simulink model "Drone_Sim_clean"  (R2018b)
settings: Solver=ode15s  StartTime=0.0  StopTime=50  FixedStep=0.1
model workspace (MAT data in the model file):
  A_matrix = [0  0  0  0  0  0  1  0  0  0  0  0; 0  0  0  0  0  0  0  1  0  0  0  0; 0  0  0  0  0  0  0  0  1  0  0  0; 0  0  0  0  0  0  0  0  0  1  0  0; 0  0  0  0  0  0  0  0  0  0  1  0; 0  0  0  0  0  0  0  0  0  0  0  1; 0  0  0  0  9.81  0  0  0  0  0  0  0; 0  0  0  0  0  -9.81  0  0  0  0  0  0; 0  0  0  0  0  0  0  0  0  0  0  0; 0  0  0  0  0  0  0  0  0  0  0  0; 0  0  0  0  0  0  0  0  0  0  0  0; 0  0  0  0  0  0  0  0  0  0  0  0]
values from neighbouring files (symbols this model uses):
  A = [ 0 0 0 0 0 0 1 0 0 0 0 0 ... (first row only)    [A_and_B_for_drone_system_dynamics_simulink.m]
  B = we .* [ 0 0 0 0 ... (first row only)    [A_and_B_for_drone_system_dynamics_simulink.m]
  C = eye(12)    [A_and_B_for_drone_system_dynamics_simulink.m]
  D = zeros(12,4)    [A_and_B_for_drone_system_dynamics_simulink.m]
libraries: simulink x7
settings Model: EnablePacing=on  Creator=harry  LastModifiedBy=Chris

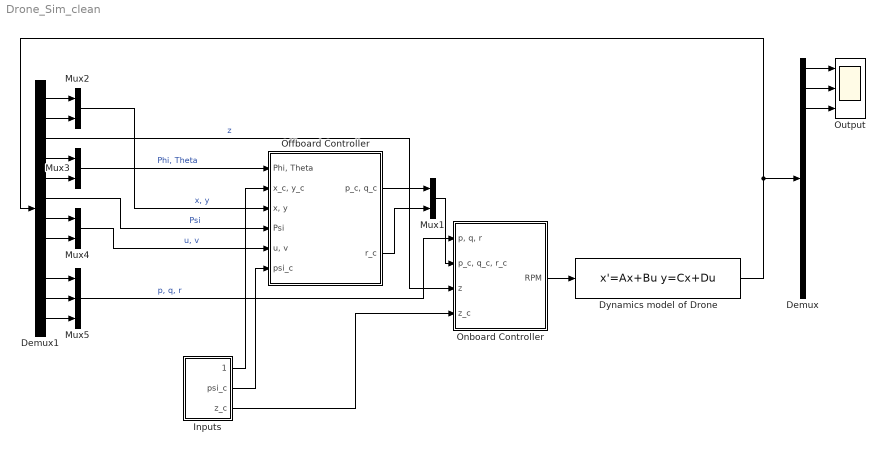
== system Drone_Sim_clean ==
  Demux : Demux  Outputs=12
  Demux1 : Demux  Outputs=12
  Dynamics model of Drone : StateSpace  A=A  B=B  C=C  D=D  InitialCondition=[0,0,0,0,0,0,0,0,0,0,0,0]  ContinuousStateAttributes='X.Y.Z.Roll.PItch.Yaw.U.V.W.Roll_Rate.Pitch_Rate.Yaw_Rate'
  Inputs : Subsystem
  Mux{1..4} (4 alike) : Mux  Inputs=2
  Mux5 : Mux  Inputs=3
  Offboard Controller : Subsystem
  Onboard Controller : Subsystem
  Output : Scope  NumInputPorts=3
  wires:
  Demux1/1 -> Mux2/1
  Demux1/2 -> Mux2/2
  Demux1/5 -> Mux3/2
  Demux1/6 -> Offboard Controller/4(Psi)  "Psi"
  Demux1/7 -> Mux4/1
  Demux1/8 -> Mux4/2
  Demux1/12 -> Mux5/3
  Demux1/11 -> Mux5/2
  Demux1/10 -> Mux5/1
  Demux/2 -> Output/2
  Mux2/1 -> Offboard Controller/3("x, y ")  "x, y"
  Mux3/1 -> Offboard Controller/1("Phi, Theta")  "Phi, Theta"
  Demux1/4 -> Mux3/1
  Mux4/1 -> Offboard Controller/5("u, v ")  "u, v"
  Inputs/1("x_c, y_c") -> Offboard Controller/2("x_c, y_c")
  Inputs/2(psi_c) -> Offboard Controller/6(psi_c)
  Offboard Controller/1("p_c, q_c") -> Mux1/1
  Offboard Controller/2(r_c) -> Mux1/2
  Mux5/1 -> Onboard Controller/1("p, q, r")  "p, q, r"
  Demux1/3 -> Onboard Controller/3(z)  "z"
  Mux1/1 -> Onboard Controller/2("p_c, q_c, r_c")
  Inputs/3(z_c) -> Onboard Controller/4(z_c)
  Onboard Controller/1(RPM) -> Dynamics model of Drone/1
  Dynamics model of Drone/1 -> Demux/1, Demux1/1
  Demux/1 -> Output/1
  Demux/3 -> Output/3

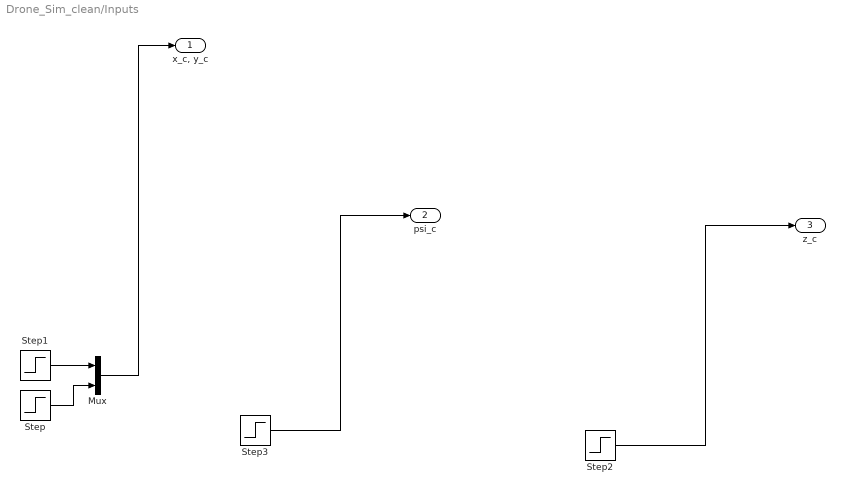
== system Drone_Sim_clean/Inputs ==
  Mux : Mux  Inputs=2
  Step : Step  After=0.3  SampleTime=0
  Step1 : Step  After=0.3  SampleTime=0
  Step2 : Step  After=0.3  SampleTime=0
  Step3 : Step  After=0  SampleTime=0
  "x_c, y_c" : Outport
  psi_c : Outport  Port=2
  z_c : Outport  Port=3
  wires:
  Step1/1 -> Mux/1
  Step2/1 -> z_c/1
  Step3/1 -> psi_c/1
  Mux/1 -> "x_c, y_c"/1
  Step/1 -> Mux/2

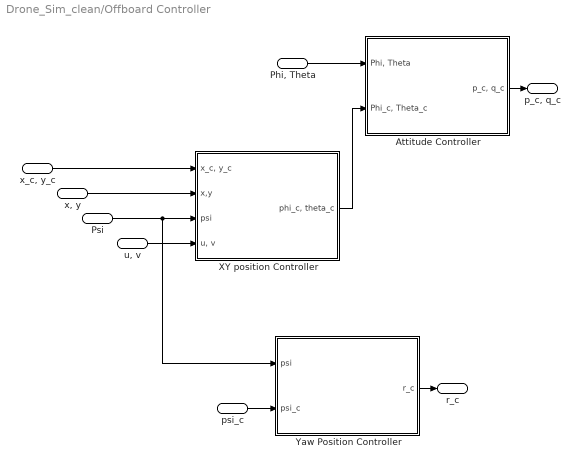
== system Drone_Sim_clean/Offboard Controller ==
  "Phi, Theta" : Inport
  "x_c, y_c" : Inport  Port=2
  "x, y " : Inport  Port=3
  Psi : Inport  Port=4
  "u, v " : Inport  Port=5
  psi_c : Inport  Port=6
  Attitude Controller : Subsystem
  XY position Controller : Subsystem
  "Yaw Position Controller " : Subsystem
  "p_c, q_c" : Outport
  r_c : Outport  Port=2
  wires:
  "u, v "/1 -> XY position Controller/4("u, v")
  "Yaw Position Controller "/1(r_c) -> r_c/1
  XY position Controller/1("phi_c, theta_c") -> Attitude Controller/2("Phi_c, Theta_c")
  Attitude Controller/1("p_c, q_c") -> "p_c, q_c"/1
  "x, y "/1 -> XY position Controller/2(x,y)
  "Phi, Theta"/1 -> Attitude Controller/1("Phi, Theta")
  "x_c, y_c"/1 -> XY position Controller/1("x_c, y_c")
  psi_c/1 -> "Yaw Position Controller "/2(psi_c)
  Psi/1 -> "Yaw Position Controller "/1(psi), XY position Controller/3(psi)

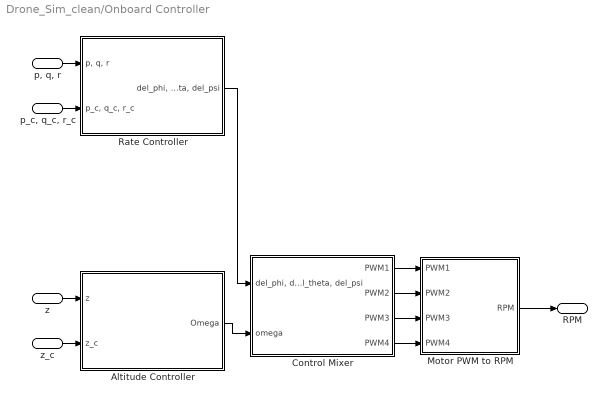
== system Drone_Sim_clean/Onboard Controller ==
  "p, q, r" : Inport
  "p_c, q_c, r_c" : Inport  Port=2
  z : Inport  Port=3
  z_c : Inport  Port=4
  Altitude Controller : Subsystem
  Control Mixer : Subsystem
  Motor PWM to RPM : Subsystem
  Rate Controller : Subsystem
  RPM : Outport
  wires:
  z_c/1 -> Altitude Controller/2(z_c)
  "p_c, q_c, r_c"/1 -> Rate Controller/2("p_c, q_c, r_c")
  Control Mixer/1("PWM1 ") -> Motor PWM to RPM/1(PWM1)
  "p, q, r"/1 -> Rate Controller/1("p, q, r")
  z/1 -> Altitude Controller/1(z)
  Motor PWM to RPM/1("RPM ") -> RPM/1
  Rate Controller/1("del_phi, del_theta, del_psi") -> Control Mixer/1("del_phi, del_theta, del_psi")
  Control Mixer/2("PWM2 ") -> Motor PWM to RPM/2(PWM2)
  Control Mixer/3(PWM3) -> Motor PWM to RPM/3(PWM3)
  Control Mixer/4("PWM4 ") -> Motor PWM to RPM/4("PWM4 ")
  Altitude Controller/1(Omega) -> Control Mixer/2("omega ")

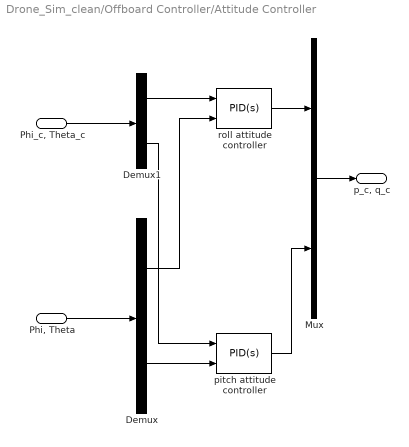
== system Drone_Sim_clean/Offboard Controller/Attitude Controller ==
  "Phi, Theta" : Inport
  "Phi_c, Theta_c" : Inport  Port=2
  Demux : Demux  Outputs=2
  Demux1 : Demux  Outputs=2
  Mux : Mux  Inputs=2
  pitch attitude controller : simulink/Continuous/PID Controller (2DOF)  Controller=PID  Form=Parallel  TimeDomain=Continuous-time  SampleTime=-1  IntegratorMethod=Forward Euler  FilterMethod=Forward Euler  ControllerParametersSource=internal  P=3.5  I=2  D=0  UseFilter=on  N=100  b=1  c=1  TunerSelectOption=Transfer Function Based (PID Tuner App)  InitialConditionSource=internal  InitialConditionForIntegrator=0  InitialConditionForFilter=0  DifferentiatorICPrevScaledInput=0  ExternalReset=none  TrackingMode=off  Kt=1  LimitOutput=on  UpperSaturationLimit=0.5  LowerSaturationLimit=-0.5  LinearizeAsGain=off  AntiWindupMode=clamping  Kb=1  POutMin=[]  POutMax=[]  IOutMin=[]  IOutMax=[]  DOutMin=[]  DOutMax=[]  NOutMin=[]  NOutMax=[]  bOutMin=[]  bOutMax=[]  cOutMin=[]  cOutMax=[]  SumOutMin=[]  SumOutMax=[]  SaturationOutMin=[]  SaturationOutMax=[]  PParamMin=[]  PParamMax=[]  IParamMin=[]  IParamMax=[]  DParamMin=[]  DParamMax=[]  NParamMin=[]  NParamMax=[]  bParamMin=[]  bParamMax=[]  cParamMin=[]  cParamMax=[]  KbParamMin=[]  KbParamMax=[]  KtParamMin=[]  KtParamMax=[]  KbOutMin=[]  KbOutMax=[]  KtOutMin=[]  KtOutMax=[]  IntegratorOutMin=[]  IntegratorOutMax=[]  FilterOutMin=[]  FilterOutMax=[]  SumI1OutMin=[]  SumI1OutMax=[]  SumI2OutMin=[]  SumI2OutMax=[]  SumI3OutMin=[]  SumI3OutMax=[]  SumI4OutMin=[]  SumI4OutMax=[]  SumDOutMin=[]  SumDOutMax=[]  Sum1OutMin=[]  Sum1OutMax=[]  Sum2OutMin=[]  Sum2OutMax=[]  Sum3OutMin=[]  Sum3OutMax=[]  DifferentiatorOutMin=[]  DifferentiatorOutMax=[]  FilterDiffOutCoefMin=[]  FilterDiffOutCoefMax=[]  ReciprocalOutMin=[]  ReciprocalOutMax=[]  SumDenOutMin=[]  SumDenOutMax=[]  SumNumOutMin=[]  SumNumOutMax=[]  DivideOutMin=[]  DivideOutMax=[]  IntegratorContinuousStateAttributes=''  IntegratorStateMustResolveToSignalObject=off  IntegratorRTWStateStorageClass=Auto  FilterContinuousStateAttributes=''  FilterStateMustResolveToSignalObject=off  FilterRTWStateStorageClass=Auto  ParallelPVariant=InternalParameters  IdealPVariant=Disabled  IVariant=InternalParameters  DVariant=InternalParameters  bVariant=InternalParameters  cVariant=InternalParameters  IntegratorVariant=Continuous  SatVariant=Enabled  AWVariant=ContClampingParallel  PCopyVariant=Disabled  TRVariant=Disabled  FdbkBlocksVariant=Forward  IdealPFdbkVariant=Disabled  SatFdbkVariant=Disabled  DerivativeFilterVariant=ContFilter  NVariant=InternalParameters  NCopyVariant=Disabled  FilterICVariant=InternalICsFilter  IntegratorICVariant=InternalICs  ExternalResetVariant=Disabled  TRSumVariant=Passthrough  SumFdbkVariant=Disabled  SumVariant=Sum_PID
  roll attitude controller : simulink/Continuous/PID Controller (2DOF)  Controller=PID  Form=Parallel  TimeDomain=Continuous-time  SampleTime=-1  IntegratorMethod=Forward Euler  FilterMethod=Forward Euler  ControllerParametersSource=internal  P=3.5  I=2  D=0  UseFilter=on  N=100  b=1  c=1  TunerSelectOption=Transfer Function Based (PID Tuner App)  InitialConditionSource=internal  InitialConditionForIntegrator=0  InitialConditionForFilter=0  DifferentiatorICPrevScaledInput=0  ExternalReset=none  TrackingMode=off  Kt=1  LimitOutput=on  UpperSaturationLimit=0.5  LowerSaturationLimit=-0.5  LinearizeAsGain=off  AntiWindupMode=clamping  Kb=1  POutMin=[]  POutMax=[]  IOutMin=[]  IOutMax=[]  DOutMin=[]  DOutMax=[]  NOutMin=[]  NOutMax=[]  bOutMin=[]  bOutMax=[]  cOutMin=[]  cOutMax=[]  SumOutMin=[]  SumOutMax=[]  SaturationOutMin=[]  SaturationOutMax=[]  PParamMin=[]  PParamMax=[]  IParamMin=[]  IParamMax=[]  DParamMin=[]  DParamMax=[]  NParamMin=[]  NParamMax=[]  bParamMin=[]  bParamMax=[]  cParamMin=[]  cParamMax=[]  KbParamMin=[]  KbParamMax=[]  KtParamMin=[]  KtParamMax=[]  KbOutMin=[]  KbOutMax=[]  KtOutMin=[]  KtOutMax=[]  IntegratorOutMin=[]  IntegratorOutMax=[]  FilterOutMin=[]  FilterOutMax=[]  SumI1OutMin=[]  SumI1OutMax=[]  SumI2OutMin=[]  SumI2OutMax=[]  SumI3OutMin=[]  SumI3OutMax=[]  SumI4OutMin=[]  SumI4OutMax=[]  SumDOutMin=[]  SumDOutMax=[]  Sum1OutMin=[]  Sum1OutMax=[]  Sum2OutMin=[]  Sum2OutMax=[]  Sum3OutMin=[]  Sum3OutMax=[]  DifferentiatorOutMin=[]  DifferentiatorOutMax=[]  FilterDiffOutCoefMin=[]  FilterDiffOutCoefMax=[]  ReciprocalOutMin=[]  ReciprocalOutMax=[]  SumDenOutMin=[]  SumDenOutMax=[]  SumNumOutMin=[]  SumNumOutMax=[]  DivideOutMin=[]  DivideOutMax=[]  IntegratorContinuousStateAttributes=''  IntegratorStateMustResolveToSignalObject=off  IntegratorRTWStateStorageClass=Auto  FilterContinuousStateAttributes=''  FilterStateMustResolveToSignalObject=off  FilterRTWStateStorageClass=Auto  ParallelPVariant=InternalParameters  IdealPVariant=Disabled  IVariant=InternalParameters  DVariant=InternalParameters  bVariant=InternalParameters  cVariant=InternalParameters  IntegratorVariant=Continuous  SatVariant=Enabled  AWVariant=ContClampingParallel  PCopyVariant=Disabled  TRVariant=Disabled  FdbkBlocksVariant=Forward  IdealPFdbkVariant=Disabled  SatFdbkVariant=Disabled  DerivativeFilterVariant=ContFilter  NVariant=InternalParameters  NCopyVariant=Disabled  FilterICVariant=InternalICsFilter  IntegratorICVariant=InternalICs  ExternalResetVariant=Disabled  TRSumVariant=Passthrough  SumFdbkVariant=Disabled  SumVariant=Sum_PID
  "p_c, q_c" : Outport  VectorParamsAs1DForOutWhenUnconnected=off
  wires:
  "Phi, Theta"/1 -> Demux/1
  "Phi_c, Theta_c"/1 -> Demux1/1
  Mux/1 -> "p_c, q_c"/1
  Demux1/1 -> roll attitude controller/1
  Demux/1 -> roll attitude controller/2
  roll attitude controller/1 -> Mux/1
  Demux/2 -> pitch attitude controller/2
  Demux1/2 -> pitch attitude controller/1
  pitch attitude controller/1 -> Mux/2

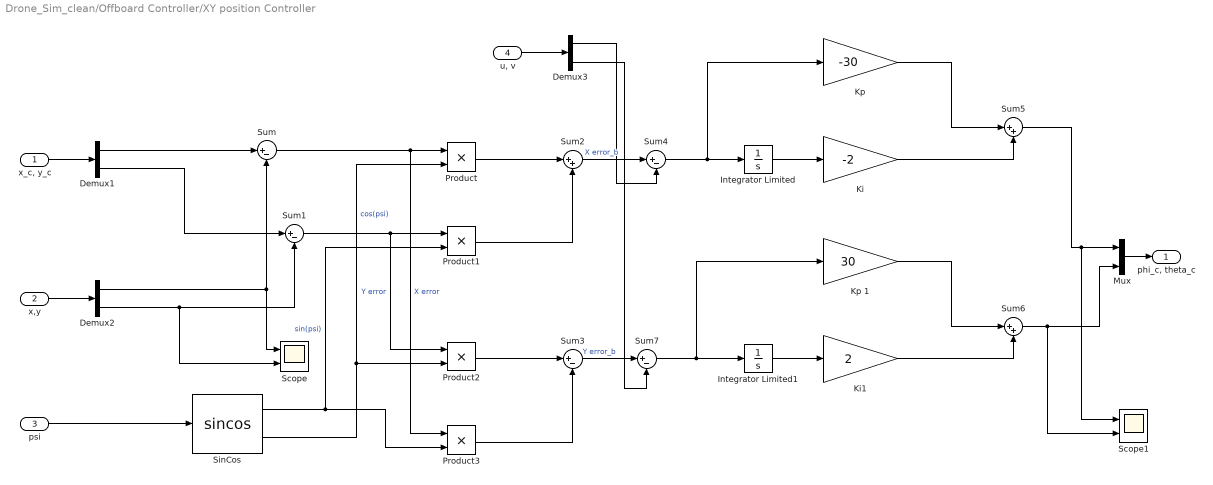
== system Drone_Sim_clean/Offboard Controller/XY position Controller ==
  "x_c, y_c" : Inport
  x,y : Inport  Port=2
  psi : Inport  Port=3
  "u, v" : Inport  Port=4
  Demux1 : Demux  Outputs=2
  Demux2 : Demux  Outputs=2
  Demux3 : Demux  Outputs=2
  Integrator Limited : Integrator  LimitOutput=on  UpperSaturationLimit=pi/6  LowerSaturationLimit=-pi/6
  Integrator Limited1 : Integrator  LimitOutput=on  UpperSaturationLimit=pi/6  LowerSaturationLimit=-pi/6
  Ki : Gain  Gain=-2
  Ki1 : Gain  Gain=2
  "Kp " : Gain  Gain=-30
  Kp 1 : Gain  Gain=30
  Mux : Mux  Inputs=2
  Product{,1..3} (4 alike) : Product
  Scope : Scope  NumInputPorts=2
  Scope1 : Scope  NumInputPorts=2
  SinCos : Trigonometry  Operator=sincos
  Sum{,1,3..4,7} (5 alike) : Sum  Inputs=|+-
  Sum2 : Sum  Inputs=|++
  Sum5 : Sum  Inputs=|++
  Sum6 : Sum  Inputs=|++
  "phi_c, theta_c" : Outport  VectorParamsAs1DForOutWhenUnconnected=off
  wires:
  "x_c, y_c"/1 -> Demux1/1
  x,y/1 -> Demux2/1
  "u, v"/1 -> Demux3/1
  Demux1/1 -> Sum/1
  Demux2/1 -> Scope/1, Sum/2
  Sum/1 -> Product3/1, Product/1  "X error"
  psi/1 -> SinCos/1
  SinCos/2 -> Product2/2, Product/2  "cos(psi)"
  Demux1/2 -> Sum1/1
  Demux2/2 -> Scope/2, Sum1/2
  Sum1/1 -> Product2/1, Product1/1  "Y error"
  SinCos/1 -> Product1/2, Product3/2  "sin(psi)"
  Product/1 -> Sum2/1
  Product1/1 -> Sum2/2
  Product2/1 -> Sum3/1
  Product3/1 -> Sum3/2
  Sum2/1 -> Sum4/1  "X error_b"
  Demux3/1 -> Sum4/2
  Sum4/1 -> "Kp "/1, Integrator Limited/1
  Integrator Limited/1 -> Ki/1
  Integrator Limited1/1 -> Ki1/1
  "Kp "/1 -> Sum5/1
  Ki/1 -> Sum5/2
  Ki1/1 -> Sum6/2
  Kp 1/1 -> Sum6/1
  Mux/1 -> "phi_c, theta_c"/1
  Sum3/1 -> Sum7/1  "Y error_b"
  Demux3/2 -> Sum7/2
  Sum7/1 -> Kp 1/1, Integrator Limited1/1
  Sum5/1 -> Scope1/1, Mux/1
  Sum6/1 -> Scope1/2, Mux/2

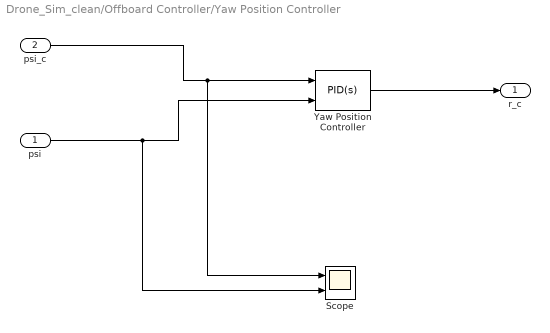
== system Drone_Sim_clean/Offboard Controller/Yaw Position Controller  ==
  psi : Inport
  psi_c : Inport  Port=2
  Scope : Scope  NumInputPorts=2
  Yaw Position Controller : simulink/Continuous/PID Controller (2DOF)  Controller=PID  Form=Parallel  TimeDomain=Continuous-time  SampleTime=-1  IntegratorMethod=Forward Euler  FilterMethod=Forward Euler  ControllerParametersSource=internal  P=3  I=0  D=0  UseFilter=on  N=100  b=1  c=1  TunerSelectOption=Transfer Function Based (PID Tuner App)  InitialConditionSource=internal  InitialConditionForIntegrator=0  InitialConditionForFilter=0  DifferentiatorICPrevScaledInput=0  ExternalReset=none  TrackingMode=off  Kt=1  LimitOutput=on  UpperSaturationLimit=1  LowerSaturationLimit=-1  LinearizeAsGain=on  AntiWindupMode=none  Kb=1  POutMin=[]  POutMax=[]  IOutMin=[]  IOutMax=[]  DOutMin=[]  DOutMax=[]  NOutMin=[]  NOutMax=[]  bOutMin=[]  bOutMax=[]  cOutMin=[]  cOutMax=[]  SumOutMin=[]  SumOutMax=[]  SaturationOutMin=[]  SaturationOutMax=[]  PParamMin=[]  PParamMax=[]  IParamMin=[]  IParamMax=[]  DParamMin=[]  DParamMax=[]  NParamMin=[]  NParamMax=[]  bParamMin=[]  bParamMax=[]  cParamMin=[]  cParamMax=[]  KbParamMin=[]  KbParamMax=[]  KtParamMin=[]  KtParamMax=[]  KbOutMin=[]  KbOutMax=[]  KtOutMin=[]  KtOutMax=[]  IntegratorOutMin=[]  IntegratorOutMax=[]  FilterOutMin=[]  FilterOutMax=[]  SumI1OutMin=[]  SumI1OutMax=[]  SumI2OutMin=[]  SumI2OutMax=[]  SumI3OutMin=[]  SumI3OutMax=[]  SumI4OutMin=[]  SumI4OutMax=[]  SumDOutMin=[]  SumDOutMax=[]  Sum1OutMin=[]  Sum1OutMax=[]  Sum2OutMin=[]  Sum2OutMax=[]  Sum3OutMin=[]  Sum3OutMax=[]  DifferentiatorOutMin=[]  DifferentiatorOutMax=[]  FilterDiffOutCoefMin=[]  FilterDiffOutCoefMax=[]  ReciprocalOutMin=[]  ReciprocalOutMax=[]  SumDenOutMin=[]  SumDenOutMax=[]  SumNumOutMin=[]  SumNumOutMax=[]  DivideOutMin=[]  DivideOutMax=[]  IntegratorContinuousStateAttributes=''  IntegratorStateMustResolveToSignalObject=off  IntegratorRTWStateStorageClass=Auto  FilterContinuousStateAttributes=''  FilterStateMustResolveToSignalObject=off  FilterRTWStateStorageClass=Auto  ParallelPVariant=InternalParameters  IdealPVariant=Disabled  IVariant=InternalParameters  DVariant=InternalParameters  bVariant=InternalParameters  cVariant=InternalParameters  IntegratorVariant=Continuous  SatVariant=Enabled  AWVariant=Passthrough  PCopyVariant=Disabled  TRVariant=Disabled  FdbkBlocksVariant=Forward  IdealPFdbkVariant=Disabled  SatFdbkVariant=Disabled  DerivativeFilterVariant=ContFilter  NVariant=InternalParameters  NCopyVariant=Disabled  FilterICVariant=InternalICsFilter  IntegratorICVariant=InternalICs  ExternalResetVariant=Disabled  TRSumVariant=Passthrough  SumFdbkVariant=Disabled  SumVariant=Sum_PID
  r_c : Outport  VectorParamsAs1DForOutWhenUnconnected=off
  wires:
  psi/1 -> Scope/2, Yaw Position Controller/2
  psi_c/1 -> Scope/1, Yaw Position Controller/1
  Yaw Position Controller/1 -> r_c/1

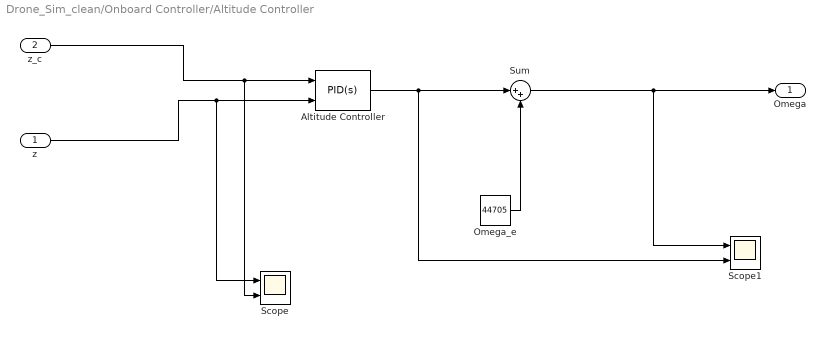
== system Drone_Sim_clean/Onboard Controller/Altitude Controller ==
  z : Inport
  z_c : Inport  Port=2
  Altitude Controller : simulink/Continuous/PID Controller (2DOF)  Controller=PID  Form=Parallel  TimeDomain=Continuous-time  SampleTime=-1  IntegratorMethod=Forward Euler  FilterMethod=Forward Euler  ControllerParametersSource=internal  P=11000  I=3500  D=9000  UseFilter=on  N=100  b=1  c=1  TunerSelectOption=Transfer Function Based (PID Tuner App)  InitialConditionSource=internal  InitialConditionForIntegrator=0  InitialConditionForFilter=0  DifferentiatorICPrevScaledInput=0  ExternalReset=none  TrackingMode=off  Kt=1  LimitOutput=on  UpperSaturationLimit=15000  LowerSaturationLimit=-20000  LinearizeAsGain=on  AntiWindupMode=clamping  Kb=1  POutMin=[]  POutMax=[]  IOutMin=[]  IOutMax=[]  DOutMin=[]  DOutMax=[]  NOutMin=[]  NOutMax=[]  bOutMin=[]  bOutMax=[]  cOutMin=[]  cOutMax=[]  SumOutMin=[]  SumOutMax=[]  SaturationOutMin=[]  SaturationOutMax=[]  PParamMin=[]  PParamMax=[]  IParamMin=[]  IParamMax=[]  DParamMin=[]  DParamMax=[]  NParamMin=[]  NParamMax=[]  bParamMin=[]  bParamMax=[]  cParamMin=[]  cParamMax=[]  KbParamMin=[]  KbParamMax=[]  KtParamMin=[]  KtParamMax=[]  KbOutMin=[]  KbOutMax=[]  KtOutMin=[]  KtOutMax=[]  IntegratorOutMin=[]  IntegratorOutMax=[]  FilterOutMin=[]  FilterOutMax=[]  SumI1OutMin=[]  SumI1OutMax=[]  SumI2OutMin=[]  SumI2OutMax=[]  SumI3OutMin=[]  SumI3OutMax=[]  SumI4OutMin=[]  SumI4OutMax=[]  SumDOutMin=[]  SumDOutMax=[]  Sum1OutMin=[]  Sum1OutMax=[]  Sum2OutMin=[]  Sum2OutMax=[]  Sum3OutMin=[]  Sum3OutMax=[]  DifferentiatorOutMin=[]  DifferentiatorOutMax=[]  FilterDiffOutCoefMin=[]  FilterDiffOutCoefMax=[]  ReciprocalOutMin=[]  ReciprocalOutMax=[]  SumDenOutMin=[]  SumDenOutMax=[]  SumNumOutMin=[]  SumNumOutMax=[]  DivideOutMin=[]  DivideOutMax=[]  IntegratorContinuousStateAttributes=''  IntegratorStateMustResolveToSignalObject=off  IntegratorRTWStateStorageClass=Auto  FilterContinuousStateAttributes=''  FilterStateMustResolveToSignalObject=off  FilterRTWStateStorageClass=Auto  ParallelPVariant=InternalParameters  IdealPVariant=Disabled  IVariant=InternalParameters  DVariant=InternalParameters  bVariant=InternalParameters  cVariant=InternalParameters  IntegratorVariant=Continuous  SatVariant=Enabled  AWVariant=ContClampingParallel  PCopyVariant=Disabled  TRVariant=Disabled  FdbkBlocksVariant=Forward  IdealPFdbkVariant=Disabled  SatFdbkVariant=Disabled  DerivativeFilterVariant=ContFilter  NVariant=InternalParameters  NCopyVariant=Disabled  FilterICVariant=InternalICsFilter  IntegratorICVariant=InternalICs  ExternalResetVariant=Disabled  TRSumVariant=Passthrough  SumFdbkVariant=Disabled  SumVariant=Sum_PID
  Omega_e : Constant  Value=44705
  Scope : Scope  NumInputPorts=2
  Scope1 : Scope  NumInputPorts=2
  Sum : Sum  Inputs=|++
  Omega : Outport  VectorParamsAs1DForOutWhenUnconnected=off
  wires:
  z_c/1 -> Scope/2, Altitude Controller/1
  Sum/1 -> Scope1/1, Omega/1
  Altitude Controller/1 -> Scope1/2, Sum/1
  Omega_e/1 -> Sum/2
  z/1 -> Scope/1, Altitude Controller/2

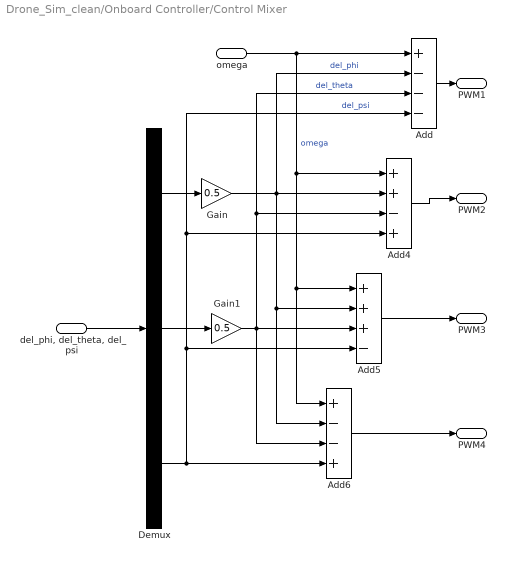
== system Drone_Sim_clean/Onboard Controller/Control Mixer ==
  "del_phi, del_theta, del_psi" : Inport
  "omega " : Inport  Port=2
  Add : Sum  Inputs=+---
  Add4 : Sum  Inputs=++-+
  Add5 : Sum  Inputs=+++-
  Add6 : Sum  Inputs=+--+
  Demux : Demux  Outputs=3
  Gain : Gain  Gain=0.5
  Gain1 : Gain  Gain=0.5
  "PWM1 " : Outport  VectorParamsAs1DForOutWhenUnconnected=off
  "PWM2 " : Outport  Port=2  VectorParamsAs1DForOutWhenUnconnected=off
  PWM3 : Outport  Port=3  VectorParamsAs1DForOutWhenUnconnected=off
  "PWM4 " : Outport  Port=4  VectorParamsAs1DForOutWhenUnconnected=off
  wires:
  "del_phi, del_theta, del_psi"/1 -> Demux/1
  Demux/1 -> Gain/1
  Demux/2 -> Gain1/1
  Add/1 -> "PWM1 "/1
  Add4/1 -> "PWM2 "/1
  Add5/1 -> PWM3/1
  Add6/1 -> "PWM4 "/1
  Demux/3 -> Add/4, Add4/4, Add5/4, Add6/4  "del_psi"
  Gain1/1 -> Add6/3, Add5/3, Add/3, Add4/3  "del_theta"
  Gain/1 -> Add/2, Add4/2, Add6/2, Add5/2  "del_phi"
  "omega "/1 -> Add/1, Add6/1, Add5/1, Add4/1  "omega"

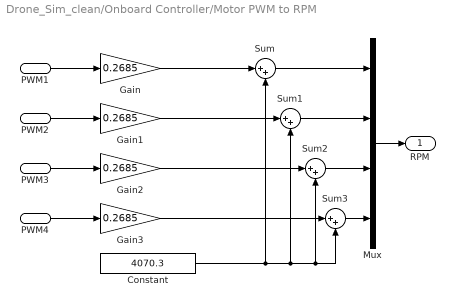
== system Drone_Sim_clean/Onboard Controller/Motor PWM to RPM ==
  PWM1 : Inport
  PWM2 : Inport  Port=2
  PWM3 : Inport  Port=3
  "PWM4 " : Inport  Port=4
  Constant : Constant  Value=4070.3
  Gain{,1..3} (4 alike) : Gain  Gain=0.2685
  Mux : Mux
  Sum{,1..3} (4 alike) : Sum  Inputs=|++
  "RPM " : Outport
  wires:
  Gain/1 -> Sum/1
  PWM1/1 -> Gain/1
  Gain1/1 -> Sum1/1
  Gain2/1 -> Sum2/1
  Gain3/1 -> Sum3/1
  PWM2/1 -> Gain1/1
  PWM3/1 -> Gain2/1
  "PWM4 "/1 -> Gain3/1
  Sum/1 -> Mux/1
  Sum1/1 -> Mux/2
  Sum2/1 -> Mux/3
  Sum3/1 -> Mux/4
  Constant/1 -> Sum/2, Sum3/2, Sum2/2, Sum1/2
  Mux/1 -> "RPM "/1

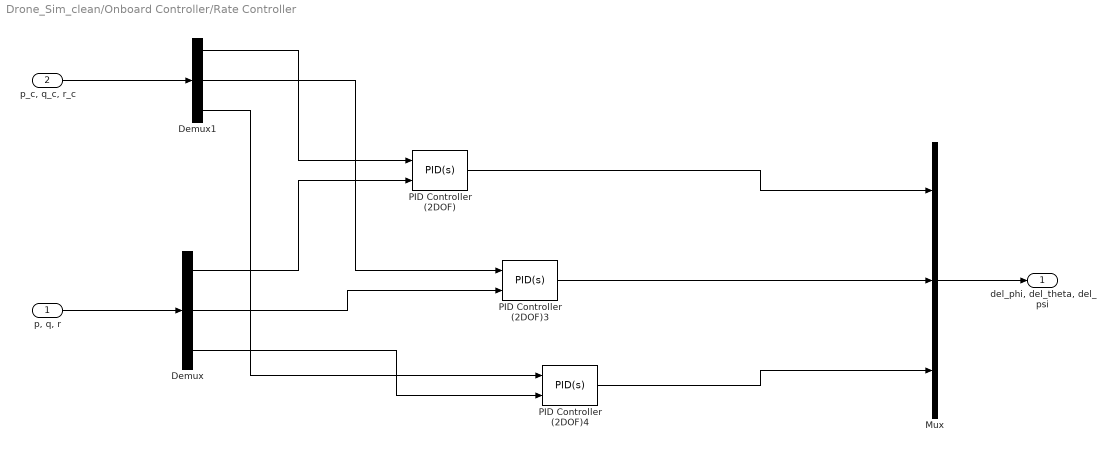
== system Drone_Sim_clean/Onboard Controller/Rate Controller ==
  "p, q, r" : Inport
  "p_c, q_c, r_c" : Inport  Port=2
  Demux : Demux  Outputs=3
  Demux1 : Demux  Outputs=3
  Mux : Mux  Inputs=3
  PID Controller (2DOF) : simulink/Continuous/PID Controller (2DOF)  Controller=PID  Form=Parallel  TimeDomain=Continuous-time  SampleTime=-1  IntegratorMethod=Forward Euler  FilterMethod=Forward Euler  ControllerParametersSource=internal  P=70  I=0  D=0  UseFilter=on  N=100  b=1  c=1  TunerSelectOption=Transfer Function Based (PID Tuner App)  InitialConditionSource=internal  InitialConditionForIntegrator=0  InitialConditionForFilter=0  DifferentiatorICPrevScaledInput=0  ExternalReset=none  TrackingMode=off  Kt=1  LimitOutput=on  UpperSaturationLimit=0.1  LowerSaturationLimit=-0.1  LinearizeAsGain=off  AntiWindupMode=clamping  Kb=1  POutMin=[]  POutMax=[]  IOutMin=[]  IOutMax=[]  DOutMin=[]  DOutMax=[]  NOutMin=[]  NOutMax=[]  bOutMin=[]  bOutMax=[]  cOutMin=[]  cOutMax=[]  SumOutMin=[]  SumOutMax=[]  SaturationOutMin=[]  SaturationOutMax=[]  PParamMin=[]  PParamMax=[]  IParamMin=[]  IParamMax=[]  DParamMin=[]  DParamMax=[]  NParamMin=[]  NParamMax=[]  bParamMin=[]  bParamMax=[]  cParamMin=[]  cParamMax=[]  KbParamMin=[]  KbParamMax=[]  KtParamMin=[]  KtParamMax=[]  KbOutMin=[]  KbOutMax=[]  KtOutMin=[]  KtOutMax=[]  IntegratorOutMin=[]  IntegratorOutMax=[]  FilterOutMin=[]  FilterOutMax=[]  SumI1OutMin=[]  SumI1OutMax=[]  SumI2OutMin=[]  SumI2OutMax=[]  SumI3OutMin=[]  SumI3OutMax=[]  SumI4OutMin=[]  SumI4OutMax=[]  SumDOutMin=[]  SumDOutMax=[]  Sum1OutMin=[]  Sum1OutMax=[]  Sum2OutMin=[]  Sum2OutMax=[]  Sum3OutMin=[]  Sum3OutMax=[]  DifferentiatorOutMin=[]  DifferentiatorOutMax=[]  FilterDiffOutCoefMin=[]  FilterDiffOutCoefMax=[]  ReciprocalOutMin=[]  ReciprocalOutMax=[]  SumDenOutMin=[]  SumDenOutMax=[]  SumNumOutMin=[]  SumNumOutMax=[]  DivideOutMin=[]  DivideOutMax=[]  IntegratorContinuousStateAttributes=''  IntegratorStateMustResolveToSignalObject=off  IntegratorRTWStateStorageClass=Auto  FilterContinuousStateAttributes=''  FilterStateMustResolveToSignalObject=off  FilterRTWStateStorageClass=Auto  ParallelPVariant=InternalParameters  IdealPVariant=Disabled  IVariant=InternalParameters  DVariant=InternalParameters  bVariant=InternalParameters  cVariant=InternalParameters  IntegratorVariant=Continuous  SatVariant=Enabled  AWVariant=ContClampingParallel  PCopyVariant=Disabled  TRVariant=Disabled  FdbkBlocksVariant=Forward  IdealPFdbkVariant=Disabled  SatFdbkVariant=Disabled  DerivativeFilterVariant=ContFilter  NVariant=InternalParameters  NCopyVariant=Disabled  FilterICVariant=InternalICsFilter  IntegratorICVariant=InternalICs  ExternalResetVariant=Disabled  TRSumVariant=Passthrough  SumFdbkVariant=Disabled  SumVariant=Sum_PID
  PID Controller (2DOF)3 : simulink/Continuous/PID Controller (2DOF)  Controller=PID  Form=Parallel  TimeDomain=Continuous-time  SampleTime=-1  IntegratorMethod=Forward Euler  FilterMethod=Forward Euler  ControllerParametersSource=internal  P=70  I=0  D=0  UseFilter=on  N=100  b=1  c=1  TunerSelectOption=Transfer Function Based (PID Tuner App)  InitialConditionSource=internal  InitialConditionForIntegrator=0  InitialConditionForFilter=0  DifferentiatorICPrevScaledInput=0  ExternalReset=none  TrackingMode=off  Kt=1  LimitOutput=on  UpperSaturationLimit=0.1  LowerSaturationLimit=-0.1  LinearizeAsGain=off  AntiWindupMode=clamping  Kb=1  POutMin=[]  POutMax=[]  IOutMin=[]  IOutMax=[]  DOutMin=[]  DOutMax=[]  NOutMin=[]  NOutMax=[]  bOutMin=[]  bOutMax=[]  cOutMin=[]  cOutMax=[]  SumOutMin=[]  SumOutMax=[]  SaturationOutMin=[]  SaturationOutMax=[]  PParamMin=[]  PParamMax=[]  IParamMin=[]  IParamMax=[]  DParamMin=[]  DParamMax=[]  NParamMin=[]  NParamMax=[]  bParamMin=[]  bParamMax=[]  cParamMin=[]  cParamMax=[]  KbParamMin=[]  KbParamMax=[]  KtParamMin=[]  KtParamMax=[]  KbOutMin=[]  KbOutMax=[]  KtOutMin=[]  KtOutMax=[]  IntegratorOutMin=[]  IntegratorOutMax=[]  FilterOutMin=[]  FilterOutMax=[]  SumI1OutMin=[]  SumI1OutMax=[]  SumI2OutMin=[]  SumI2OutMax=[]  SumI3OutMin=[]  SumI3OutMax=[]  SumI4OutMin=[]  SumI4OutMax=[]  SumDOutMin=[]  SumDOutMax=[]  Sum1OutMin=[]  Sum1OutMax=[]  Sum2OutMin=[]  Sum2OutMax=[]  Sum3OutMin=[]  Sum3OutMax=[]  DifferentiatorOutMin=[]  DifferentiatorOutMax=[]  FilterDiffOutCoefMin=[]  FilterDiffOutCoefMax=[]  ReciprocalOutMin=[]  ReciprocalOutMax=[]  SumDenOutMin=[]  SumDenOutMax=[]  SumNumOutMin=[]  SumNumOutMax=[]  DivideOutMin=[]  DivideOutMax=[]  IntegratorContinuousStateAttributes=''  IntegratorStateMustResolveToSignalObject=off  IntegratorRTWStateStorageClass=Auto  FilterContinuousStateAttributes=''  FilterStateMustResolveToSignalObject=off  FilterRTWStateStorageClass=Auto  ParallelPVariant=InternalParameters  IdealPVariant=Disabled  IVariant=InternalParameters  DVariant=InternalParameters  bVariant=InternalParameters  cVariant=InternalParameters  IntegratorVariant=Continuous  SatVariant=Enabled  AWVariant=ContClampingParallel  PCopyVariant=Disabled  TRVariant=Disabled  FdbkBlocksVariant=Forward  IdealPFdbkVariant=Disabled  SatFdbkVariant=Disabled  DerivativeFilterVariant=ContFilter  NVariant=InternalParameters  NCopyVariant=Disabled  FilterICVariant=InternalICsFilter  IntegratorICVariant=InternalICs  ExternalResetVariant=Disabled  TRSumVariant=Passthrough  SumFdbkVariant=Disabled  SumVariant=Sum_PID
  PID Controller (2DOF)4 : simulink/Continuous/PID Controller (2DOF)  Controller=PID  Form=Parallel  TimeDomain=Continuous-time  SampleTime=-1  IntegratorMethod=Forward Euler  FilterMethod=Forward Euler  ControllerParametersSource=internal  P=70  I=16.70  D=0  UseFilter=on  N=100  b=1  c=1  TunerSelectOption=Transfer Function Based (PID Tuner App)  InitialConditionSource=internal  InitialConditionForIntegrator=0  InitialConditionForFilter=0  DifferentiatorICPrevScaledInput=0  ExternalReset=none  TrackingMode=off  Kt=1  LimitOutput=on  UpperSaturationLimit=0.1  LowerSaturationLimit=-0.1  LinearizeAsGain=off  AntiWindupMode=clamping  Kb=1  POutMin=[]  POutMax=[]  IOutMin=[]  IOutMax=[]  DOutMin=[]  DOutMax=[]  NOutMin=[]  NOutMax=[]  bOutMin=[]  bOutMax=[]  cOutMin=[]  cOutMax=[]  SumOutMin=[]  SumOutMax=[]  SaturationOutMin=[]  SaturationOutMax=[]  PParamMin=[]  PParamMax=[]  IParamMin=[]  IParamMax=[]  DParamMin=[]  DParamMax=[]  NParamMin=[]  NParamMax=[]  bParamMin=[]  bParamMax=[]  cParamMin=[]  cParamMax=[]  KbParamMin=[]  KbParamMax=[]  KtParamMin=[]  KtParamMax=[]  KbOutMin=[]  KbOutMax=[]  KtOutMin=[]  KtOutMax=[]  IntegratorOutMin=[]  IntegratorOutMax=[]  FilterOutMin=[]  FilterOutMax=[]  SumI1OutMin=[]  SumI1OutMax=[]  SumI2OutMin=[]  SumI2OutMax=[]  SumI3OutMin=[]  SumI3OutMax=[]  SumI4OutMin=[]  SumI4OutMax=[]  SumDOutMin=[]  SumDOutMax=[]  Sum1OutMin=[]  Sum1OutMax=[]  Sum2OutMin=[]  Sum2OutMax=[]  Sum3OutMin=[]  Sum3OutMax=[]  DifferentiatorOutMin=[]  DifferentiatorOutMax=[]  FilterDiffOutCoefMin=[]  FilterDiffOutCoefMax=[]  ReciprocalOutMin=[]  ReciprocalOutMax=[]  SumDenOutMin=[]  SumDenOutMax=[]  SumNumOutMin=[]  SumNumOutMax=[]  DivideOutMin=[]  DivideOutMax=[]  IntegratorContinuousStateAttributes=''  IntegratorStateMustResolveToSignalObject=off  IntegratorRTWStateStorageClass=Auto  FilterContinuousStateAttributes=''  FilterStateMustResolveToSignalObject=off  FilterRTWStateStorageClass=Auto  ParallelPVariant=InternalParameters  IdealPVariant=Disabled  IVariant=InternalParameters  DVariant=InternalParameters  bVariant=InternalParameters  cVariant=InternalParameters  IntegratorVariant=Continuous  SatVariant=Enabled  AWVariant=ContClampingParallel  PCopyVariant=Disabled  TRVariant=Disabled  FdbkBlocksVariant=Forward  IdealPFdbkVariant=Disabled  SatFdbkVariant=Disabled  DerivativeFilterVariant=ContFilter  NVariant=InternalParameters  NCopyVariant=Disabled  FilterICVariant=InternalICsFilter  IntegratorICVariant=InternalICs  ExternalResetVariant=Disabled  TRSumVariant=Passthrough  SumFdbkVariant=Disabled  SumVariant=Sum_PID
  "del_phi, del_theta, del_psi" : Outport  VectorParamsAs1DForOutWhenUnconnected=off
  wires:
  "p, q, r"/1 -> Demux/1
  "p_c, q_c, r_c"/1 -> Demux1/1
  Mux/1 -> "del_phi, del_theta, del_psi"/1
  Demux1/1 -> PID Controller (2DOF)/1
  Demux/1 -> PID Controller (2DOF)/2
  Demux1/2 -> PID Controller (2DOF)3/1
  Demux/2 -> PID Controller (2DOF)3/2
  Demux1/3 -> PID Controller (2DOF)4/1
  Demux/3 -> PID Controller (2DOF)4/2
  PID Controller (2DOF)/1 -> Mux/1
  PID Controller (2DOF)3/1 -> Mux/2
  PID Controller (2DOF)4/1 -> Mux/3
